simulink library "miniMUTT_Aero_Lib"  (Simulink 8.0)
settings: Solver=ode45  StartTime=0.0  StopTime=10.0  RelTol=1e-3
values from neighbouring files (symbols this model uses):
  AC = miniMUTT_config    [UAV_config.m]    (also in UAV_modelconfig.mat = )
  TrimCondition =     [UAV_trimcondition.mat]
undefined symbols (not defined in the file or in its folder): full
libraries: simulink x1
settings Model: Creator=austinmurch  LastModifiedBy=hpfifer

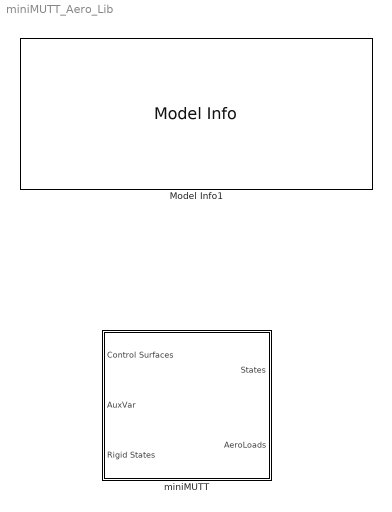
== system miniMUTT_Aero_Lib ==
  Model Info1 : simulink/Model-Wide Utilities/Model Info  InitialBlockCM=None  BlockCM=None  Frame=on  DisplayStringWithTags=|  HorizontalTextAlignment=Left  LeftAlignmentValue=0.02  SourceBlockDiagram=miniMUTT_Aero_Lib  TagMaxNumber=20
      | MODEL INFORMATION
      | mini MUTT aircraft Aerodynamic Model Library
      | 
      | University of Minnesota
      | Aerospace Engineering and Mechanics
      | Copyright 2011 Regents of the University of Minnesota. All rights reserved.
      | 
      | == SVN Info ==
      | %<ModelVersion>
      | Last modified by %<LastModifiedBy> on %<LastModificationDate>
  miniMUTT : Subsystem

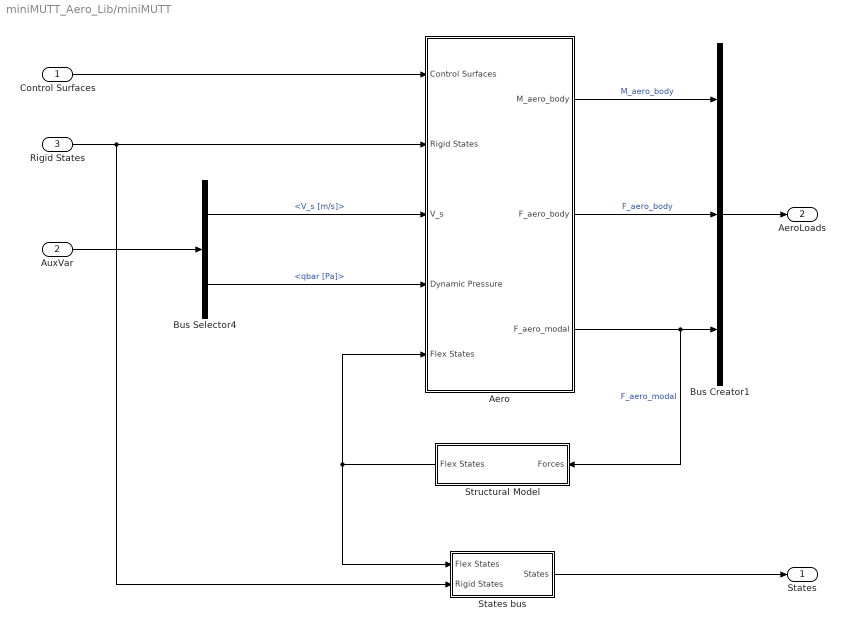
== system miniMUTT_Aero_Lib/miniMUTT ==
  Control Surfaces : Inport
  AuxVar : Inport  Port=2
  Rigid States : Inport  Port=3
  Aero : Subsystem  mask{RFA=AC.Aero.RFA, c_ref=AC.Geometry.c, DT1_omega=AC.Aero.DT1_omega, nh=0, nf=0, nx2=[], DT1_Vel_ConSurf=0, DT2_Acc_AllMode=0}
      mask prompts: RFA "RFA Data Structure"
      mask help:
      | Realize a RFA of
      | [P_b;P_f] = RFA * [u_x2; u_b; u_f; du_b; d_uf]
      mask init:
      | % Get Size
      | nh = size(RFA.A0,1);
      | nb = 6;
      | nf = nh-nb;
      | nx2 = size(RFA.A0,2)-nh;
      | 
      | % Define DT1
      | DT1_Vel_ConSurf = ss(tf([DT1_omega,0], [1,DT1_omega]))*eye(nx2);
      | DT1_Acc_AllModes = ss(tf([DT1_omega,0], [1,DT1_omega]))*eye(nh+nx2);
      | 
      | % ConSurf_dis = c2d(DT1_Vel_ConSurf,0.02);
      | % AllMode_dis = c2d(DT2_Acc_AllMode,0.02);
      | % 
      | % [ConSurf_dis_num ConSurf_dis_den] = ss2tf(ConSurf_dis.a,ConSurf_dis.b,ConSurf_dis.c,ConSurf_dis.d);
      | % [AllMode_dis_num AllMode_dis_den] = ss2tf(AllMode_dis.a,AllMode_dis.b,AllMode_dis.c,AllMode_dis.d);
  Bus Creator1 : BusCreator  Inputs=3
  Bus Selector4 : BusSelector  OutputSignals=WindAxesParam.V_s [m/s],qbar [Pa]
  States bus : Subsystem
  Structural Model : Subsystem
  States : Outport
  AeroLoads : Outport  Port=2
  wires:
  Bus Selector4/2 -> Aero/4(Dynamic Pressure)  "<qbar [Pa]>"
  Bus Selector4/1 -> Aero/3(V_s)  "<V_s [m/s]>"
  Bus Creator1/1 -> AeroLoads/1
  Structural Model/1(Flex States) -> Aero/5(Flex States), States bus/1(Flex States)
  Aero/3(F_aero_modal) -> Structural Model/1(Forces), Bus Creator1/3  "F_aero_modal"
  Aero/1(M_aero_body) -> Bus Creator1/1  "M_aero_body"
  Aero/2(F_aero_body) -> Bus Creator1/2  "F_aero_body"
  AuxVar/1 -> Bus Selector4/1
  Rigid States/1 -> States bus/2(Rigid States), Aero/2(Rigid States)
  Control Surfaces/1 -> Aero/1(Control Surfaces)
  States bus/1(States) -> States/1

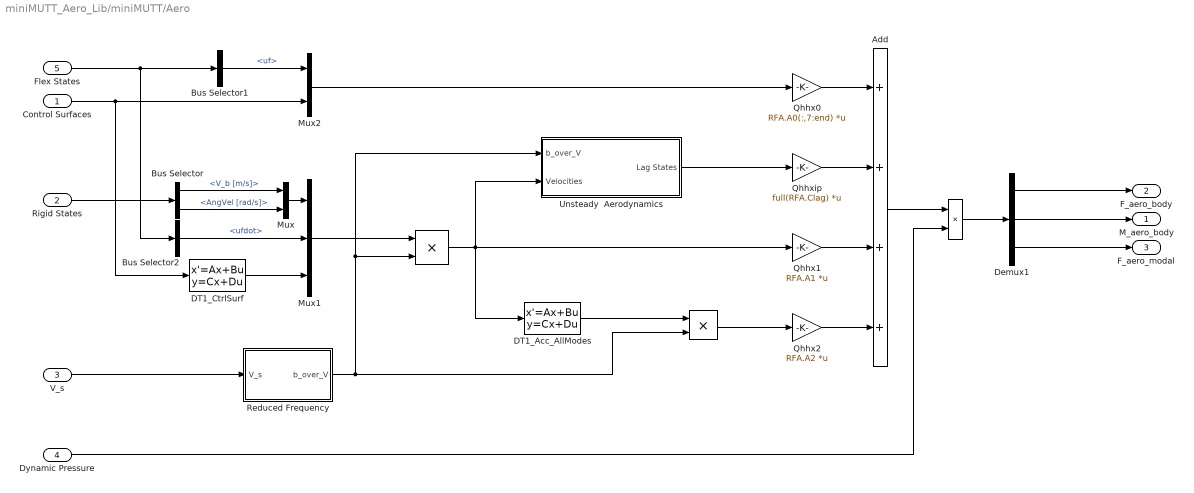
== system miniMUTT_Aero_Lib/miniMUTT/Aero ==
  Control Surfaces : Inport
  Rigid States : Inport  Port=2
  V_s : Inport  Port=3
  Dynamic Pressure : Inport  Port=4
  Flex States : Inport  Port=5
  "   " : Product  RndMeth=Zero
  "    " : Product  RndMeth=Zero
  "      " : Product  RndMeth=Zero
  Add : Sum  Inputs=++++
  Bus Selector : BusSelector  OutputSignals=V_b [m/s],AngVel [rad/s]
  Bus Selector1 : BusSelector  OutputSignals=uf
  Bus Selector2 : BusSelector  OutputSignals=ufdot
  DT1_Acc_AllModes : StateSpace  A=DT1_Acc_AllModes.a  B=DT1_Acc_AllModes.b  C=DT1_Acc_AllModes.c  D=DT1_Acc_AllModes.d  X0=TrimCondition.DT1AccAllModes
  DT1_CtrlSurf : StateSpace  A=DT1_Vel_ConSurf.a  B=DT1_Vel_ConSurf.b  C=DT1_Vel_ConSurf.c  D=DT1_Vel_ConSurf.d  X0=TrimCondition.DT1CtrlSurfIni
  Demux1 : Demux  Outputs=[3,3,-1]
  Mux : Mux  Inputs=2
  Mux1 : Mux  Inputs=3
  Mux2 : Mux  Inputs=2
  Qhhx0 : Gain  Gain=RFA.A0(:,7:end)  Multiplication=Matrix(K*u)
  Qhhx1 : Gain  Gain=RFA.A1  Multiplication=Matrix(K*u)
  Qhhx2 : Gain  Gain=RFA.A2  Multiplication=Matrix(K*u)
  Qhhxip : Gain  Gain=full(RFA.Clag)  Multiplication=Matrix(K*u)
  Reduced Frequency : Subsystem
  Unsteady  Aerodynamics : Subsystem
  M_aero_body : Outport
  F_aero_body : Outport  Port=2
  F_aero_modal : Outport  Port=3
  wires:
  Unsteady  Aerodynamics/1(Lag States) -> Qhhxip/1
  Bus Selector2/1 -> Mux1/2  "<ufdot>"
  Bus Selector1/1 -> Mux2/1  "<uf>"
  Flex States/1 -> Bus Selector1/1, Bus Selector2/1
  Mux/1 -> Mux1/1
  Bus Selector/2 -> Mux/2  "<AngVel [rad/s]>"
  Bus Selector/1 -> Mux/1  "<V_b [m/s]>"
  Demux1/3 -> F_aero_modal/1
  Demux1/2 -> M_aero_body/1
  Demux1/1 -> F_aero_body/1
  "    "/1 -> Demux1/1
  Qhhx0/1 -> Add/1
  Rigid States/1 -> Bus Selector/1
  Control Surfaces/1 -> DT1_CtrlSurf/1, Mux2/2
  V_s/1 -> Reduced Frequency/1(V_s)
  Mux2/1 -> Qhhx0/1
  Add/1 -> "    "/1
  Dynamic Pressure/1 -> "    "/2
  "   "/1 -> Qhhx2/1
  "      "/1 -> DT1_Acc_AllModes/1, Qhhx1/1, Unsteady  Aerodynamics/2(Velocities)
  Reduced Frequency/1(b_over_V) -> Unsteady  Aerodynamics/1(b_over_V), "      "/2, "   "/2
  Mux1/1 -> "      "/1
  Qhhxip/1 -> Add/2
  Qhhx1/1 -> Add/3
  Qhhx2/1 -> Add/4
  DT1_CtrlSurf/1 -> Mux1/3
  DT1_Acc_AllModes/1 -> "   "/1

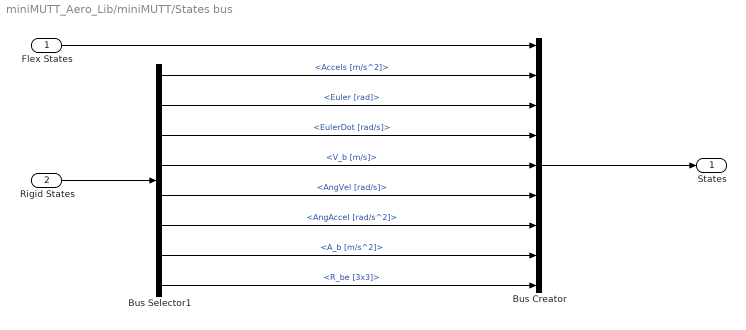
== system miniMUTT_Aero_Lib/miniMUTT/States bus ==
  Flex States : Inport
  Rigid States : Inport  Port=2
  Bus Creator : BusCreator  Inputs=9
  Bus Selector1 : BusSelector  OutputSignals=Accels [m/s^2],Euler [rad],EulerDot [rad/s],V_b [m/s],AngVel [rad/s],AngAccel [rad/s^2],A_b [m/s^2],R_be [3x3]
  States : Outport
  wires:
  Bus Creator/1 -> States/1
  Rigid States/1 -> Bus Selector1/1
  Flex States/1 -> Bus Creator/1
  Bus Selector1/1 -> Bus Creator/2  "<Accels [m/s^2]>"
  Bus Selector1/7 -> Bus Creator/8  "<A_b [m/s^2]>"
  Bus Selector1/3 -> Bus Creator/4  "<EulerDot [rad/s]>"
  Bus Selector1/2 -> Bus Creator/3  "<Euler [rad]>"
  Bus Selector1/4 -> Bus Creator/5  "<V_b [m/s]>"
  Bus Selector1/8 -> Bus Creator/9  "<R_be [3x3]>"
  Bus Selector1/5 -> Bus Creator/6  "<AngVel [rad/s]>"
  Bus Selector1/6 -> Bus Creator/7  "<AngAccel [rad/s^2]>"

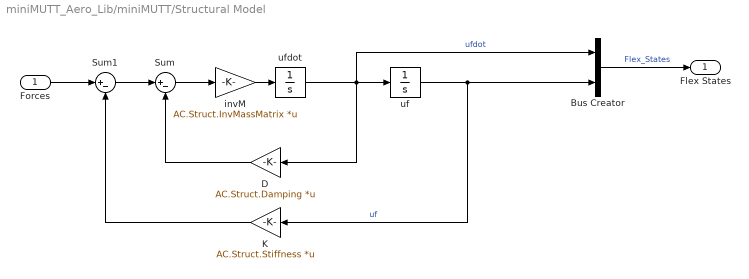
== system miniMUTT_Aero_Lib/miniMUTT/Structural Model ==
  Forces : Inport
  Bus Creator : BusCreator  Inputs=2
  D : Gain  Gain=AC.Struct.Damping  Multiplication=Matrix(K*u)
  K : Gain  Gain=AC.Struct.Stiffness  Multiplication=Matrix(K*u)
  Sum : Sum  Inputs=|+-
  Sum1 : Sum  Inputs=|+-
  invM : Gain  Gain=AC.Struct.InvMassMatrix  Multiplication=Matrix(K*u)
  uf : Integrator  InitialCondition=TrimCondition.FlexIni
  ufdot : Integrator  InitialCondition=TrimCondition.FlexRatesIni
  Flex States : Outport
  wires:
  Bus Creator/1 -> Flex States/1  "Flex_States"
  K/1 -> Sum1/2
  Sum1/1 -> Sum/1
  D/1 -> Sum/2
  Sum/1 -> invM/1
  invM/1 -> ufdot/1
  uf/1 -> K/1, Bus Creator/2  "uf"
  ufdot/1 -> uf/1, D/1, Bus Creator/1  "ufdot"
  Forces/1 -> Sum1/1

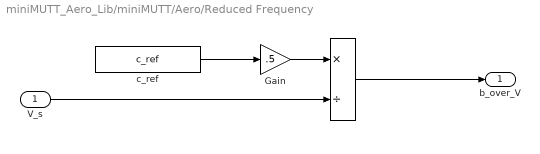
== system miniMUTT_Aero_Lib/miniMUTT/Aero/Reduced Frequency ==
  V_s : Inport
  "     " : Product  Inputs=*/
  Gain : Gain  Gain=.5
  c_ref : Constant  Value=c_ref
  b_over_V : Outport
  wires:
  c_ref/1 -> Gain/1
  Gain/1 -> "     "/1
  V_s/1 -> "     "/2
  "     "/1 -> b_over_V/1

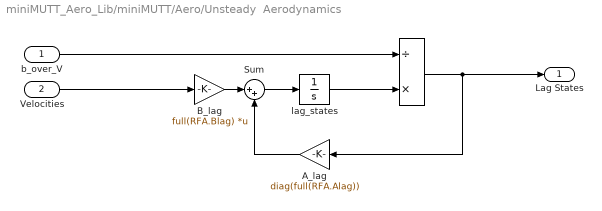
== system miniMUTT_Aero_Lib/miniMUTT/Aero/Unsteady  Aerodynamics ==
  b_over_V : Inport
  Velocities : Inport  Port=2
  "    " : Product  Inputs=/*
  A_lag : Gain  Gain=diag(full(RFA.Alag))
  B_lag : Gain  Gain=full(RFA.Blag)  Multiplication=Matrix(K*u)
  Sum : Sum  Inputs=|++
  lag_states : Integrator  InitialCondition=TrimCondition.LagStatesIni
  Lag States : Outport
  wires:
  b_over_V/1 -> "    "/1
  Velocities/1 -> B_lag/1
  B_lag/1 -> Sum/1
  Sum/1 -> lag_states/1
  A_lag/1 -> Sum/2
  lag_states/1 -> "    "/2
  "    "/1 -> A_lag/1, Lag States/1
